simulink model "testing_m_function"  (R2024a)
settings: Solver=FixedStepAuto  StartTime=0.0  StopTime=10.0  FixedStep=0.01  RelTol=1e-3
undefined symbols (not defined in the file or in its folder): q0, vec
libraries: sharedtransform x5
settings Model: Creator=bemran  LastModifiedBy=bemran

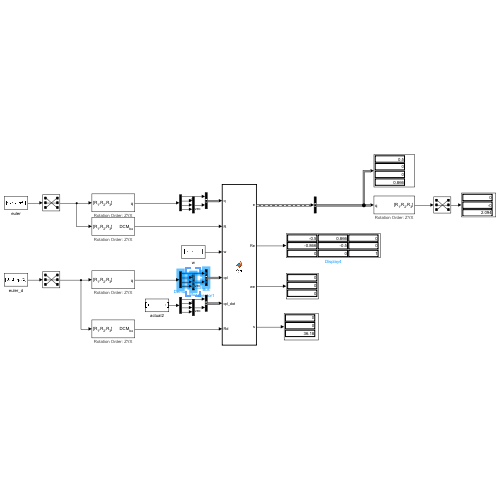
[thumbnail: Simulink's stored preview of the top-level diagram]
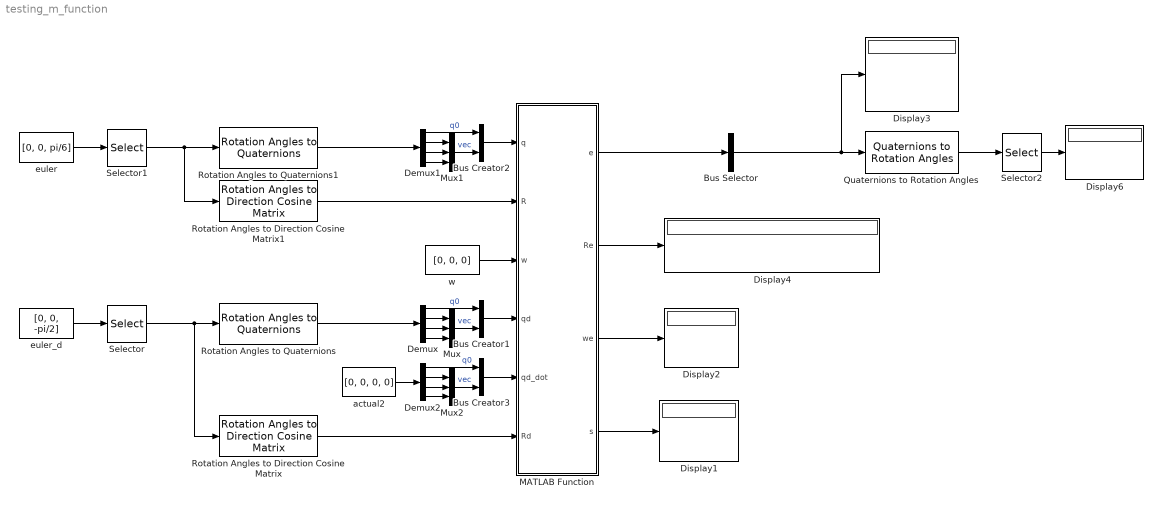
== system testing_m_function ==
  Bus Creator1 : BusCreator  Inputs=q0,vec  OutDataTypeStr=Bus: QuaturnionBus
  Bus Creator2 : BusCreator  Inputs=q0,vec  OutDataTypeStr=Bus: QuaturnionBus
  Bus Creator3 : BusCreator  Inputs=q0,vec  OutDataTypeStr=Bus: QuaturnionBus
  Bus Selector : BusSelector  OutputSignals=q0,vec  OutputAsBus=on
  Demux : Demux
  Demux1 : Demux
  Demux2 : Demux
  Display{1..4,6} (5 alike) : Display
  MATLAB Function : MATLAB Function  TreatAsAtomicUnit=on
  Mux : Mux  Inputs=3
  Mux1 : Mux  Inputs=3
  Mux2 : Mux  Inputs=3
  Quaternions to Rotation Angles : sharedtransform/Quaternions to Rotation Angles  rotationOrder=ZYX  aMode=aMode
  Rotation Angles to Direction Cosine Matrix : sharedtransform/Rotation Angles to Direction Cosine Matrix  rotationOrder=ZYX  aMode=aMode
  Rotation Angles to Direction Cosine Matrix1 : sharedtransform/Rotation Angles to Direction Cosine Matrix  rotationOrder=ZYX  aMode=aMode
  Rotation Angles to Quaternions : sharedtransform/Rotation Angles to Quaternions  rotationOrder=ZYX  aMode=aMode
  Rotation Angles to Quaternions1 : sharedtransform/Rotation Angles to Quaternions  rotationOrder=ZYX  aMode=aMode
  Selector : Selector  InputPortWidth=3  IndexOptions=Index vector (dialog)  Indices=[3 2 1]  OutputSizes=1
  Selector1 : Selector  InputPortWidth=3  IndexOptions=Index vector (dialog)  Indices=[3 2 1]  OutputSizes=1
  Selector2 : Selector  InputPortWidth=3  IndexOptions=Index vector (dialog)  Indices=[3 2 1]  OutputSizes=1
  actual2 : Constant  Value=[0, 0, 0, 0]
  euler : Constant  Value=[0, 0, pi/6]
  euler_d : Constant  Value=[0, 0, -pi/2]
  w : Constant  Value=[0, 0, 0]
  wires:
  euler_d/1 -> Selector/1
  euler/1 -> Selector1/1
  Selector1/1 -> Rotation Angles to Quaternions1/1, Rotation Angles to Direction Cosine Matrix1/1
  Selector/1 -> Rotation Angles to Direction Cosine Matrix/1, Rotation Angles to Quaternions/1
  Rotation Angles to Quaternions/1 -> Demux/1
  Demux/2 -> Mux/1
  Demux/3 -> Mux/2
  Demux/4 -> Mux/3
  Mux/1 -> Bus Creator1/2  "vec"
  Demux/1 -> Bus Creator1/1  "q0"
  Mux1/1 -> Bus Creator2/2  "vec"
  Demux1/1 -> Bus Creator2/1  "q0"
  Demux1/2 -> Mux1/1
  Demux1/3 -> Mux1/2
  Demux1/4 -> Mux1/3
  Rotation Angles to Quaternions1/1 -> Demux1/1
  Rotation Angles to Direction Cosine Matrix/1 -> MATLAB Function/6(Rd)
  Bus Creator2/1 -> MATLAB Function/1(q)
  Bus Creator1/1 -> MATLAB Function/4(qd)
  MATLAB Function/1(e) -> Bus Selector/1
  MATLAB Function/2(Re) -> Display4/1
  Bus Selector/1 -> Quaternions to Rotation Angles/1, Display3/1
  Rotation Angles to Direction Cosine Matrix1/1 -> MATLAB Function/2(R)
  Quaternions to Rotation Angles/1 -> Selector2/1
  Selector2/1 -> Display6/1
  Demux2/1 -> Bus Creator3/1  "q0"
  Mux2/1 -> Bus Creator3/2  "vec"
  Demux2/4 -> Mux2/3
  Demux2/3 -> Mux2/2
  Demux2/2 -> Mux2/1
  Bus Creator3/1 -> MATLAB Function/5(qd_dot)
  w/1 -> MATLAB Function/3(w)
  actual2/1 -> Demux2/1
  MATLAB Function/4(s) -> Display1/1
  MATLAB Function/3(we) -> Display2/1

== matlab function testing_m_function/MATLAB Function ==
  data: q input Bus: QuaturnionBus size=1; R input size=[3 3]; w input size=[1 3]; qd input Bus: QuaturnionBus size=1; qd_dot input Bus: QuaturnionBus; Rd input size=[3 3]; e output Bus: QuaturnionBus size=1; Re output size=[3 3]; we output size=[1 3]; s output
function [e, Re, we, s] = fcn(q, R, w, qd, qd_dot, Rd)

e.q0 = qd.q0 * q.q0 + qd.vec * q.vec';
e.vec = qd.q0 * q.vec - q.q0 * qd.vec + cross(q.vec, qd.vec);
Re = R*Rd';

wd = qd_dot.vec / (qd.q0*eye(3) + Skew(qd.vec));
we = w - wd * Re';
e0_dot = 0.5 * e.vec * we';
evec_dot = 0.5 * (e.q0 * we + cross(e.vec, we));

% parameters
gama1 = 10;
gama2 = 30;
gama3 = 1;
n = 3;
l = 5;
pow = n/l;
eps = 0.01;

de = DeltaE(e.vec, pow ,eps);
s = evec_dot + gama1 * e.vec + gama2 * de + gama3 * we;

function de = DeltaE (e, pow, eps)
    de = e;
    for i = 1:3
        if abs(e(i)) > eps
            de(i) = e(i)^pow;
        end
    end
end

function y = Skew(v)
    y = [    0,  -v(3),  v(2);...
          v(3),      0, -v(1);...
         -v(2),   v(1),    0];
end
end
